simulink model "offboard_SSC_simscape"  (R2025b)
settings: Solver=ode23t  StartTime=0.0  StopTime=0.5  RelTol=1e-3
undefined symbols (not defined in the file): PLL_3ph__class, V_ref
libraries: fl_lib x43, nesl_utility x23, ee_lib x9, simulink x6, eeTransforms x2, batteryecm_lib x1, eeSinusoidalMeasurement x1
(part 2 of 2)

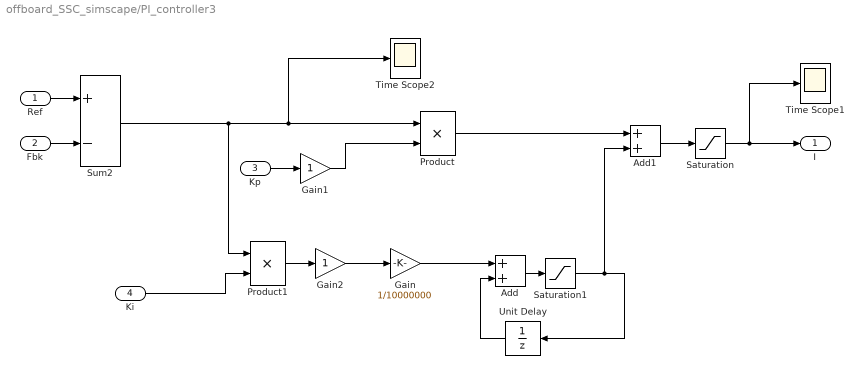
== system offboard_SSC_simscape/PI_controller3 ==
  Ref : Inport
  Fbk : Inport  Port=2
  Kp : Inport  Port=3
  Ki : Inport  Port=4
  Add : Sum
  Add1 : Sum
  Gain : Gain  Gain=1/10000000
  Gain1 : Gain
  Gain2 : Gain
  Product : Product  OutDataTypeStr=Inherit: Same as first input
  Product1 : Product  OutDataTypeStr=Inherit: Same as first input
  Saturation : Saturate  UpperLimit=50  LowerLimit=-50  LinearizeAsGain=off  ZeroCross=off
  Saturation1 : Saturate  UpperLimit=50  LowerLimit=-50  LinearizeAsGain=off  ZeroCross=off
  Sum2 : Sum  Inputs=+-
  Time Scope1 : Scope
      settings: TimeUnits=Metric (based on Time Span)  ActiveDisplayYMinimum=10.50458  ActiveDisplayYMaximum=21.05505  YLabel=Amplitude  DataLoggingVariableName=ScopeData5
  Time Scope2 : Scope
      settings: TimeUnits=Metric (based on Time Span)  ActiveDisplayYMinimum=-48.22028  ActiveDisplayYMaximum=227.58003  YLabel=Amplitude  DataLoggingVariableName=ScopeData6
  Unit Delay : UnitDelay  InitialCondition=0.9  SampleTime=-1  HasFrameUpgradeWarning=on
  I : Outport
  wires:
  Fbk/1 -> Sum2/2
  Ref/1 -> Sum2/1
  Product1/1 -> Gain2/1
  Product/1 -> Add1/1
  Gain/1 -> Add/1
  Unit Delay/1 -> Add/2
  Ki/1 -> Product1/2
  Gain2/1 -> Gain/1
  Add1/1 -> Saturation/1
  Saturation/1 -> Time Scope1/1, I/1
  Kp/1 -> Gain1/1
  Gain1/1 -> Product/2
  Sum2/1 -> Product1/1, Time Scope2/1, Product/1
  Add/1 -> Saturation1/1
  Saturation1/1 -> Add1/2, Unit Delay/1

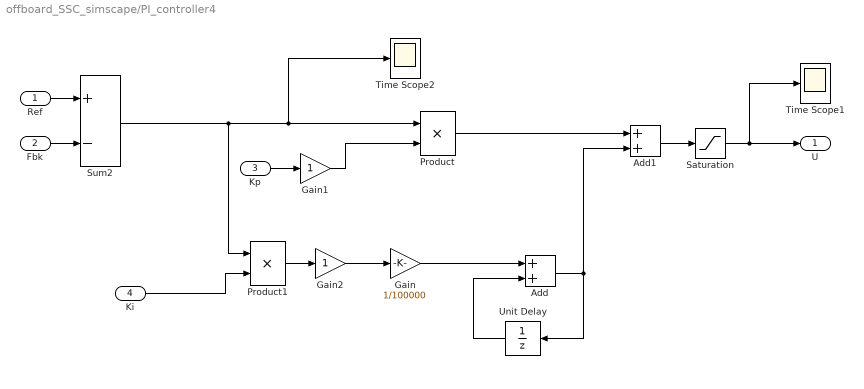
== system offboard_SSC_simscape/PI_controller4 ==
  Ref : Inport
  Fbk : Inport  Port=2
  Kp : Inport  Port=3
  Ki : Inport  Port=4
  Add : Sum
  Add1 : Sum
  Gain : Gain  Gain=1/100000
  Gain1 : Gain
  Gain2 : Gain
  Product : Product  OutDataTypeStr=Inherit: Same as first input
  Product1 : Product  OutDataTypeStr=Inherit: Same as first input
  Saturation : Saturate  UpperLimit=400  LowerLimit=-400  LinearizeAsGain=off  ZeroCross=off
  Sum2 : Sum  Inputs=+-
  Time Scope1 : Scope
      settings: TimeUnits=Metric (based on Time Span)  ActiveDisplayYMinimum=-500  ActiveDisplayYMaximum=500  YLabel=Amplitude  DataLoggingVariableName=ScopeData5
  Time Scope2 : Scope
      settings: TimeUnits=Metric (based on Time Span)  ActiveDisplayYMinimum=-48.22028  ActiveDisplayYMaximum=227.58003  YLabel=Amplitude  DataLoggingVariableName=ScopeData6
  Unit Delay : UnitDelay  SampleTime=-1  HasFrameUpgradeWarning=on
  U : Outport
  wires:
  Fbk/1 -> Sum2/2
  Ref/1 -> Sum2/1
  Product1/1 -> Gain2/1
  Add/1 -> Unit Delay/1, Add1/2
  Product/1 -> Add1/1
  Gain/1 -> Add/1
  Unit Delay/1 -> Add/2
  Ki/1 -> Product1/2
  Gain2/1 -> Gain/1
  Add1/1 -> Saturation/1
  Saturation/1 -> Time Scope1/1, U/1
  Kp/1 -> Gain1/1
  Gain1/1 -> Product/2
  Sum2/1 -> Product1/1, Time Scope2/1, Product/1

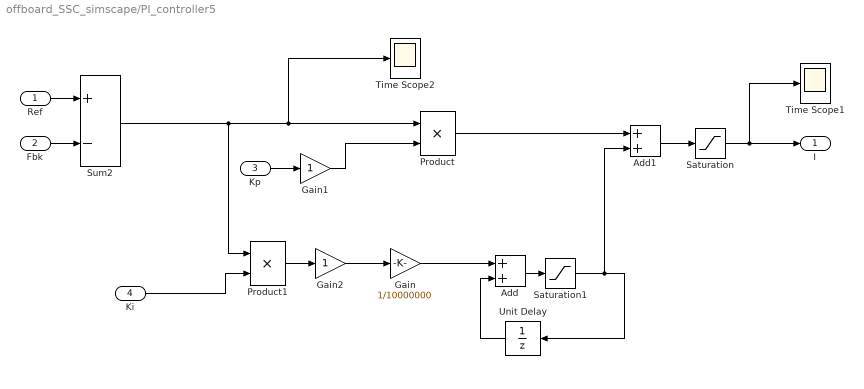
== system offboard_SSC_simscape/PI_controller5 ==
  Ref : Inport
  Fbk : Inport  Port=2
  Kp : Inport  Port=3
  Ki : Inport  Port=4
  Add : Sum
  Add1 : Sum
  Gain : Gain  Gain=1/10000000
  Gain1 : Gain
  Gain2 : Gain
  Product : Product  OutDataTypeStr=Inherit: Same as first input
  Product1 : Product  OutDataTypeStr=Inherit: Same as first input
  Saturation : Saturate  UpperLimit=50  LowerLimit=0  LinearizeAsGain=off  ZeroCross=off
  Saturation1 : Saturate  UpperLimit=50  LowerLimit=-50  LinearizeAsGain=off  ZeroCross=off
  Sum2 : Sum  Inputs=+-
  Time Scope1 : Scope
      settings: TimeUnits=Metric (based on Time Span)  ActiveDisplayYMinimum=10.50458  ActiveDisplayYMaximum=21.05505  YLabel=Amplitude  DataLoggingVariableName=ScopeData5
  Time Scope2 : Scope
      settings: TimeUnits=Metric (based on Time Span)  ActiveDisplayYMinimum=-48.22028  ActiveDisplayYMaximum=227.58003  YLabel=Amplitude  DataLoggingVariableName=ScopeData6
  Unit Delay : UnitDelay  InitialCondition=0.9  SampleTime=-1  HasFrameUpgradeWarning=on
  I : Outport
  wires:
  Fbk/1 -> Sum2/2
  Ref/1 -> Sum2/1
  Product1/1 -> Gain2/1
  Product/1 -> Add1/1
  Gain/1 -> Add/1
  Unit Delay/1 -> Add/2
  Ki/1 -> Product1/2
  Gain2/1 -> Gain/1
  Add1/1 -> Saturation/1
  Saturation/1 -> Time Scope1/1, I/1
  Kp/1 -> Gain1/1
  Gain1/1 -> Product/2
  Sum2/1 -> Product1/1, Time Scope2/1, Product/1
  Add/1 -> Saturation1/1
  Saturation1/1 -> Add1/2, Unit Delay/1

== system offboard_SSC_simscape/PLL (3ph) ==
  abc : Inport
  "Sinusoidal Measurement (PLL, Three-Phase)" : eeSinusoidalMeasurement/Sinusoidal Measurement (PLL, Three-Phase)  Kp_LF=180  Ki_LF=3200  F0=60  Theta0=PLL_3ph__class([0 60]).objParamMappingDerived.NewDerivedParam.Theta0  Ts=0.0001
  Terminator : Terminator
  Freq : Outport  VectorParamsAs1DForOutWhenUnconnected=off
  wt : Outport  Port=2  VectorParamsAs1DForOutWhenUnconnected=off
  wires:
  "Sinusoidal Measurement (PLL, Three-Phase)"/3 -> Terminator/1
  "Sinusoidal Measurement (PLL, Three-Phase)"/2 -> wt/1
  "Sinusoidal Measurement (PLL, Three-Phase)"/1 -> Freq/1
  abc/1 -> "Sinusoidal Measurement (PLL, Three-Phase)"/1

== system offboard_SSC_simscape/Subsystem ==
  PS-Simulink Converter2 : nesl_utility/PS-Simulink Converter  PhysicalDomain=network_engine_domain  SubClassName=ps_output  LeftPortType=input  RightPortType=output  PseudoPeriodic=off  Frequencies=[]  VectorFormat=inherit  Unit=inherit  AffineConversion=off
  Unit Delay1 : UnitDelay  SampleTime=-1  HasFrameUpgradeWarning=on
  Voltage Sensor : fl_lib/Electrical/Electrical Sensors/Voltage Sensor
  + : PMIOPort  Side=Left
  - : PMIOPort  Port=2  Side=Right
  V : Outport
  wires:
  PS-Simulink Converter2/1 -> Unit Delay1/1
  Unit Delay1/1 -> V/1
  connections:
  Voltage Sensor/LConn1 -- +/RConn1
  PS-Simulink Converter2/LConn1 -- Voltage Sensor/RConn1
  Voltage Sensor/RConn2 -- -/RConn1

== system offboard_SSC_simscape/Subsystem1 ==
  Va : Inport
  Va1 : Inport  Port=2
  Add1 : Sum
  Constant8 : Constant  Value=0.5
  Divide : Product  Inputs=*/
  Logical Operator1 : Logic  Operator=NOT  AllPortsSameDT=off  OutDataTypeStr=boolean
  Relational Operator : RelationalOperator  OutDataTypeStr=boolean  ZeroCross=off  InputSameDT=off
  Repeating Sequence : simulink/Sources/Repeating Sequence  rep_seq_t=[0 1/30000/2 1/30000]  rep_seq_y=[0 1 0]
  Scope1 : Scope  NumInputPorts=2
      settings: ActiveDisplayYMinimum=-0.12496  ActiveDisplayYMaximum=1.12466  DataLoggingVariableName=ScopeData3
  Scope2 : Scope  NumInputPorts=2
      settings: ActiveDisplayYMinimum=-0.59999  ActiveDisplayYMaximum=3.15933
  Scope3 : Scope  NumInputPorts=2
      settings: ActiveDisplayYMinimum=-0.125  ActiveDisplayYMaximum=1.125  DataLoggingVariableName=ScopeData2
  Vcomp*2 : Constant  Value=1200
  A : Outport
  A' : Outport  Port=2
  wires:
  Va/1 -> Divide/1
  Divide/1 -> Add1/1
  Add1/1 -> Scope2/1, Relational Operator/2
  Constant8/1 -> Add1/2
  Repeating Sequence/1 -> Scope1/1, Relational Operator/1
  Logical Operator1/1 -> Scope3/1, A/1
  Relational Operator/1 -> Scope3/2, A'/1, Logical Operator1/1
  Va1/1 -> Divide/2

== system offboard_SSC_simscape/Subsystem2 ==
  Vb : Inport
  Va : Inport  Port=2
  Add1 : Sum
  Constant8 : Constant  Value=0.5
  Divide : Product  Inputs=*/
  Logical Operator1 : Logic  Operator=NOT  AllPortsSameDT=off  OutDataTypeStr=boolean
  Relational Operator : RelationalOperator  OutDataTypeStr=boolean  ZeroCross=off  InputSameDT=off
  Repeating Sequence : simulink/Sources/Repeating Sequence  rep_seq_t=[0 1/30000/2 1/30000]  rep_seq_y=[0 1 0]
  Scope1 : Scope  NumInputPorts=2
      settings: ActiveDisplayYMinimum=-0.125  ActiveDisplayYMaximum=1.125  DataLoggingVariableName=ScopeData3
  Scope4 : Scope  NumInputPorts=2
      settings: ActiveDisplayYMinimum=-500  ActiveDisplayYMaximum=500  DataLoggingVariableName=ScopeData3
  Vcomp*2 : Constant  Value=1200
  B : Outport
  B' : Outport  Port=2
  wires:
  Vb/1 -> Divide/1
  Divide/1 -> Add1/1
  Add1/1 -> Relational Operator/2, Scope4/2
  Constant8/1 -> Add1/2
  Repeating Sequence/1 -> Scope1/1, Relational Operator/1
  Logical Operator1/1 -> B/1
  Relational Operator/1 -> B'/1, Logical Operator1/1
  Va/1 -> Divide/2

== system offboard_SSC_simscape/Subsystem3 ==
  Va : Inport
  Add1 : Sum
  Constant8 : Constant  Value=0.5
  Divide : Product  Inputs=*/
  Logical Operator1 : Logic  Operator=NOT  AllPortsSameDT=off  OutDataTypeStr=boolean
  Relational Operator : RelationalOperator  OutDataTypeStr=boolean  ZeroCross=off  InputSameDT=off
  Repeating Sequence : simulink/Sources/Repeating Sequence  rep_seq_t=[0 1/100000/2 1/100000]  rep_seq_y=[0 1 0]
  Scope1 : Scope  NumInputPorts=2
      settings: ActiveDisplayYMinimum=-0.12496  ActiveDisplayYMaximum=1.12466  DataLoggingVariableName=ScopeData3
  Scope2 : Scope  NumInputPorts=2
      settings: ActiveDisplayYMinimum=-0.59999  ActiveDisplayYMaximum=3.15933
  Scope3 : Scope  NumInputPorts=2
      settings: ActiveDisplayYMinimum=-0.125  ActiveDisplayYMaximum=1.125  DataLoggingVariableName=ScopeData2
  Vcomp*2 : Constant  Value=800
  A : Outport
  A' : Outport  Port=2
  wires:
  Va/1 -> Divide/1
  Divide/1 -> Add1/1
  Add1/1 -> Scope2/1, Relational Operator/2
  Constant8/1 -> Add1/2
  Repeating Sequence/1 -> Scope1/1, Relational Operator/1
  Logical Operator1/1 -> Scope3/1, A/1
  Relational Operator/1 -> Scope3/2, A'/1, Logical Operator1/1
  Vcomp*2/1 -> Divide/2

== system offboard_SSC_simscape/Subsystem4 ==
  Vc : Inport
  Va : Inport  Port=2
  Add1 : Sum
  Constant8 : Constant  Value=0.5
  Divide : Product  Inputs=*/
  Logical Operator1 : Logic  Operator=NOT  AllPortsSameDT=off  OutDataTypeStr=boolean
  Relational Operator : RelationalOperator  OutDataTypeStr=boolean  ZeroCross=off  InputSameDT=off
  Repeating Sequence : simulink/Sources/Repeating Sequence  rep_seq_t=[0 1/30000/2 1/30000]  rep_seq_y=[0 1 0]
  Scope1 : Scope  NumInputPorts=2
      settings: ActiveDisplayYMinimum=-0.125  ActiveDisplayYMaximum=1.125  DataLoggingVariableName=ScopeData3
  Scope4 : Scope  NumInputPorts=2
      settings: ActiveDisplayYMinimum=-500  ActiveDisplayYMaximum=500  DataLoggingVariableName=ScopeData3
  Vcomp*2 : Constant  Value=1200
  C : Outport
  C' : Outport  Port=2
  wires:
  Vc/1 -> Divide/1
  Divide/1 -> Add1/1
  Add1/1 -> Relational Operator/2, Scope4/2
  Constant8/1 -> Add1/2
  Repeating Sequence/1 -> Scope1/1, Relational Operator/1
  Logical Operator1/1 -> C/1
  Relational Operator/1 -> C'/1, Logical Operator1/1
  Va/1 -> Divide/2

== system offboard_SSC_simscape/Subsystem5 ==
  Va : Inport
  Add1 : Sum
  Constant8 : Constant  Value=0.5
  Divide : Product  Inputs=*/
  Logical Operator1 : Logic  Operator=NOT  AllPortsSameDT=off  OutDataTypeStr=boolean
  Relational Operator : RelationalOperator  OutDataTypeStr=boolean  ZeroCross=off  InputSameDT=off
  Repeating Sequence : simulink/Sources/Repeating Sequence  rep_seq_t=[0 1/100000/2 1/100000]  rep_seq_y=[0 1 0]
  Scope1 : Scope  NumInputPorts=2
      settings: ActiveDisplayYMinimum=-0.12496  ActiveDisplayYMaximum=1.12466  DataLoggingVariableName=ScopeData3
  Scope2 : Scope  NumInputPorts=2
      settings: ActiveDisplayYMinimum=-0.59999  ActiveDisplayYMaximum=3.15933
  Scope3 : Scope  NumInputPorts=2
      settings: ActiveDisplayYMinimum=-0.125  ActiveDisplayYMaximum=1.125  DataLoggingVariableName=ScopeData2
  Vcomp*2 : Constant  Value=800
  A : Outport
  A' : Outport  Port=2
  wires:
  Va/1 -> Divide/1
  Divide/1 -> Add1/1
  Add1/1 -> Scope2/1, Relational Operator/2
  Constant8/1 -> Add1/2
  Repeating Sequence/1 -> Scope1/1, Relational Operator/1
  Logical Operator1/1 -> Scope3/1, A/1
  Relational Operator/1 -> Scope3/2, A'/1, Logical Operator1/1
  Vcomp*2/1 -> Divide/2

== system offboard_SSC_simscape/Subsystem6 ==
  Va : Inport
  Add1 : Sum
  Constant8 : Constant  Value=0.5
  Divide : Product  Inputs=*/
  Logical Operator1 : Logic  Operator=NOT  AllPortsSameDT=off  OutDataTypeStr=boolean
  Relational Operator : RelationalOperator  OutDataTypeStr=boolean  ZeroCross=off  InputSameDT=off
  Repeating Sequence : simulink/Sources/Repeating Sequence  rep_seq_t=[0 1/100000/2 1/100000]  rep_seq_y=[0 1 0]
  Scope1 : Scope  NumInputPorts=2
      settings: ActiveDisplayYMinimum=-0.12496  ActiveDisplayYMaximum=1.12466  DataLoggingVariableName=ScopeData3
  Scope2 : Scope  NumInputPorts=2
      settings: ActiveDisplayYMinimum=-0.59999  ActiveDisplayYMaximum=3.15933
  Scope3 : Scope  NumInputPorts=2
      settings: ActiveDisplayYMinimum=-0.125  ActiveDisplayYMaximum=1.125  DataLoggingVariableName=ScopeData2
  Vcomp*2 : Constant  Value=800
  A : Outport
  A' : Outport  Port=2
  wires:
  Va/1 -> Divide/1
  Divide/1 -> Add1/1
  Add1/1 -> Scope2/1, Relational Operator/2
  Constant8/1 -> Add1/2
  Repeating Sequence/1 -> Scope1/1, Relational Operator/1
  Logical Operator1/1 -> Scope3/1, A/1
  Relational Operator/1 -> Scope3/2, A'/1, Logical Operator1/1
  Vcomp*2/1 -> Divide/2

== system offboard_SSC_simscape/Subsystem8 ==
  PS-Simulink Converter2 : nesl_utility/PS-Simulink Converter  PhysicalDomain=network_engine_domain  SubClassName=ps_output  LeftPortType=input  RightPortType=output  PseudoPeriodic=off  Frequencies=[]  VectorFormat=inherit  Unit=inherit  AffineConversion=off
  Unit Delay1 : UnitDelay  SampleTime=-1  HasFrameUpgradeWarning=on
  Voltage Sensor : fl_lib/Electrical/Electrical Sensors/Voltage Sensor
  + : PMIOPort  Side=Left
  - : PMIOPort  Port=2  Side=Right
  V : Outport
  wires:
  Unit Delay1/1 -> V/1
  PS-Simulink Converter2/1 -> Unit Delay1/1
  connections:
  Voltage Sensor/RConn2 -- -/RConn1
  PS-Simulink Converter2/LConn1 -- Voltage Sensor/RConn1
  Voltage Sensor/LConn1 -- +/RConn1

== system offboard_SSC_simscape/DC//DC1/S1 ==
  g : Inport
  Diode : fl_lib/Electrical/Electrical Elements/Diode  Vf=1e-3 V  Ron=1e-2 Ohm  Goff=1e-5 1/Ohm  i_specify=off  i_priority=None  i=0 A  i_nominal_specify=off  i_nominal_value=1  i_nominal_unit=A  v_specify=off  v_priority=None  v=0 V  v_nominal_specify=off  v_nominal_value=1  v_nominal_unit=V
  S1 : fl_lib/Electrical/Electrical Elements/Switch  R_closed=0.1 Ohm  G_open=1e-5 1/Ohm  Threshold=0.5  i_specify=off  i_priority=None  i=0 A  i_nominal_specify=off  i_nominal_value=1  i_nominal_unit=A  v_specify=off  v_priority=None  v=0 V  v_nominal_specify=off  v_nominal_value=1  v_nominal_unit=V
  Simulink-PS Converter : nesl_utility/Simulink-PS Converter  PhysicalDomain=network_engine_domain  SubClassName=ps_input  LeftPortType=input  RightPortType=output  PseudoPeriodic=off  Frequencies=[]  NoiseDistribution=none  NoiseParameters=[]  Unit=1  AffineConversion=off  FilteringAndDerivatives=zero  SimscapeFilterOrder=1  InputFilterTimeConstant=0.001  UdotUserProvided=0
  + : PMIOPort  Side=Left
  - : PMIOPort  Port=2  Side=Right
  wires:
  g/1 -> Simulink-PS Converter/1
  connections:
  S1/RConn2 -- -/RConn1 -- Diode/LConn1
  Diode/RConn1 -- +/RConn1 -- S1/LConn1
  Simulink-PS Converter/RConn1 -- S1/RConn1

== system offboard_SSC_simscape/DC//DC1/S2 ==
  g : Inport
  Diode : fl_lib/Electrical/Electrical Elements/Diode  Vf=1e-3 V  Ron=1e-2 Ohm  Goff=1e-5 1/Ohm  i_specify=off  i_priority=None  i=0 A  i_nominal_specify=off  i_nominal_value=1  i_nominal_unit=A  v_specify=off  v_priority=None  v=0 V  v_nominal_specify=off  v_nominal_value=1  v_nominal_unit=V
  S1 : fl_lib/Electrical/Electrical Elements/Switch  R_closed=0.1 Ohm  G_open=1e-5 1/Ohm  Threshold=0.5  i_specify=off  i_priority=None  i=0 A  i_nominal_specify=off  i_nominal_value=1  i_nominal_unit=A  v_specify=off  v_priority=None  v=0 V  v_nominal_specify=off  v_nominal_value=1  v_nominal_unit=V
  Simulink-PS Converter : nesl_utility/Simulink-PS Converter  PhysicalDomain=network_engine_domain  SubClassName=ps_input  LeftPortType=input  RightPortType=output  PseudoPeriodic=off  Frequencies=[]  NoiseDistribution=none  NoiseParameters=[]  Unit=1  AffineConversion=off  FilteringAndDerivatives=zero  SimscapeFilterOrder=1  InputFilterTimeConstant=0.001  UdotUserProvided=0
  + : PMIOPort  Side=Left
  - : PMIOPort  Port=2  Side=Right
  wires:
  g/1 -> Simulink-PS Converter/1
  connections:
  Simulink-PS Converter/RConn1 -- S1/RConn1
  S1/LConn1 -- +/RConn1 -- Diode/RConn1
  Diode/LConn1 -- -/RConn1 -- S1/RConn2

== system offboard_SSC_simscape/DC//DC2/S1 ==
  g : Inport
  Diode : fl_lib/Electrical/Electrical Elements/Diode  Vf=1e-3 V  Ron=1e-2 Ohm  Goff=1e-5 1/Ohm  i_specify=off  i_priority=None  i=0 A  i_nominal_specify=off  i_nominal_value=1  i_nominal_unit=A  v_specify=off  v_priority=None  v=0 V  v_nominal_specify=off  v_nominal_value=1  v_nominal_unit=V
  S1 : fl_lib/Electrical/Electrical Elements/Switch  R_closed=0.1 Ohm  G_open=1e-5 1/Ohm  Threshold=0.5  i_specify=off  i_priority=None  i=0 A  i_nominal_specify=off  i_nominal_value=1  i_nominal_unit=A  v_specify=off  v_priority=None  v=0 V  v_nominal_specify=off  v_nominal_value=1  v_nominal_unit=V
  Simulink-PS Converter : nesl_utility/Simulink-PS Converter  PhysicalDomain=network_engine_domain  SubClassName=ps_input  LeftPortType=input  RightPortType=output  PseudoPeriodic=off  Frequencies=[]  NoiseDistribution=none  NoiseParameters=[]  Unit=1  AffineConversion=off  FilteringAndDerivatives=zero  SimscapeFilterOrder=1  InputFilterTimeConstant=0.001  UdotUserProvided=0
  + : PMIOPort  Side=Left
  - : PMIOPort  Port=2  Side=Right
  wires:
  g/1 -> Simulink-PS Converter/1
  connections:
  S1/RConn2 -- -/RConn1 -- Diode/LConn1
  Diode/RConn1 -- +/RConn1 -- S1/LConn1
  Simulink-PS Converter/RConn1 -- S1/RConn1

== system offboard_SSC_simscape/DC//DC2/S2 ==
  g : Inport
  Diode : fl_lib/Electrical/Electrical Elements/Diode  Vf=1e-3 V  Ron=1e-2 Ohm  Goff=1e-5 1/Ohm  i_specify=off  i_priority=None  i=0 A  i_nominal_specify=off  i_nominal_value=1  i_nominal_unit=A  v_specify=off  v_priority=None  v=0 V  v_nominal_specify=off  v_nominal_value=1  v_nominal_unit=V
  S1 : fl_lib/Electrical/Electrical Elements/Switch  R_closed=0.1 Ohm  G_open=1e-5 1/Ohm  Threshold=0.5  i_specify=off  i_priority=None  i=0 A  i_nominal_specify=off  i_nominal_value=1  i_nominal_unit=A  v_specify=off  v_priority=None  v=0 V  v_nominal_specify=off  v_nominal_value=1  v_nominal_unit=V
  Simulink-PS Converter : nesl_utility/Simulink-PS Converter  PhysicalDomain=network_engine_domain  SubClassName=ps_input  LeftPortType=input  RightPortType=output  PseudoPeriodic=off  Frequencies=[]  NoiseDistribution=none  NoiseParameters=[]  Unit=1  AffineConversion=off  FilteringAndDerivatives=zero  SimscapeFilterOrder=1  InputFilterTimeConstant=0.001  UdotUserProvided=0
  + : PMIOPort  Side=Left
  - : PMIOPort  Port=2  Side=Right
  wires:
  g/1 -> Simulink-PS Converter/1
  connections:
  Simulink-PS Converter/RConn1 -- S1/RConn1
  S1/LConn1 -- +/RConn1 -- Diode/RConn1
  Diode/LConn1 -- -/RConn1 -- S1/RConn2

== system offboard_SSC_simscape/DC//DC3/S1 ==
  g : Inport
  Diode : fl_lib/Electrical/Electrical Elements/Diode  Vf=1e-3 V  Ron=1e-2 Ohm  Goff=1e-5 1/Ohm  i_specify=off  i_priority=None  i=0 A  i_nominal_specify=off  i_nominal_value=1  i_nominal_unit=A  v_specify=off  v_priority=None  v=0 V  v_nominal_specify=off  v_nominal_value=1  v_nominal_unit=V
  S1 : fl_lib/Electrical/Electrical Elements/Switch  R_closed=0.1 Ohm  G_open=1e-5 1/Ohm  Threshold=0.5  i_specify=off  i_priority=None  i=0 A  i_nominal_specify=off  i_nominal_value=1  i_nominal_unit=A  v_specify=off  v_priority=None  v=0 V  v_nominal_specify=off  v_nominal_value=1  v_nominal_unit=V
  Simulink-PS Converter : nesl_utility/Simulink-PS Converter  PhysicalDomain=network_engine_domain  SubClassName=ps_input  LeftPortType=input  RightPortType=output  PseudoPeriodic=off  Frequencies=[]  NoiseDistribution=none  NoiseParameters=[]  Unit=1  AffineConversion=off  FilteringAndDerivatives=zero  SimscapeFilterOrder=1  InputFilterTimeConstant=0.001  UdotUserProvided=0
  + : PMIOPort  Side=Left
  - : PMIOPort  Port=2  Side=Right
  wires:
  g/1 -> Simulink-PS Converter/1
  connections:
  S1/RConn2 -- -/RConn1 -- Diode/LConn1
  Diode/RConn1 -- +/RConn1 -- S1/LConn1
  Simulink-PS Converter/RConn1 -- S1/RConn1

== system offboard_SSC_simscape/DC//DC3/S2 ==
  g : Inport
  Diode : fl_lib/Electrical/Electrical Elements/Diode  Vf=1e-3 V  Ron=1e-2 Ohm  Goff=1e-5 1/Ohm  i_specify=off  i_priority=None  i=0 A  i_nominal_specify=off  i_nominal_value=1  i_nominal_unit=A  v_specify=off  v_priority=None  v=0 V  v_nominal_specify=off  v_nominal_value=1  v_nominal_unit=V
  S1 : fl_lib/Electrical/Electrical Elements/Switch  R_closed=0.1 Ohm  G_open=1e-5 1/Ohm  Threshold=0.5  i_specify=off  i_priority=None  i=0 A  i_nominal_specify=off  i_nominal_value=1  i_nominal_unit=A  v_specify=off  v_priority=None  v=0 V  v_nominal_specify=off  v_nominal_value=1  v_nominal_unit=V
  Simulink-PS Converter : nesl_utility/Simulink-PS Converter  PhysicalDomain=network_engine_domain  SubClassName=ps_input  LeftPortType=input  RightPortType=output  PseudoPeriodic=off  Frequencies=[]  NoiseDistribution=none  NoiseParameters=[]  Unit=1  AffineConversion=off  FilteringAndDerivatives=zero  SimscapeFilterOrder=1  InputFilterTimeConstant=0.001  UdotUserProvided=0
  + : PMIOPort  Side=Left
  - : PMIOPort  Port=2  Side=Right
  wires:
  g/1 -> Simulink-PS Converter/1
  connections:
  Simulink-PS Converter/RConn1 -- S1/RConn1
  S1/LConn1 -- +/RConn1 -- Diode/RConn1
  Diode/LConn1 -- -/RConn1 -- S1/RConn2

== system offboard_SSC_simscape/Front End/S1 ==
  g : Inport
  Diode : fl_lib/Electrical/Electrical Elements/Diode  Vf=1e-3 V  Ron=1e-2 Ohm  Goff=1e-5 1/Ohm  i_specify=off  i_priority=None  i=0 A  i_nominal_specify=off  i_nominal_value=1  i_nominal_unit=A  v_specify=off  v_priority=None  v=0 V  v_nominal_specify=off  v_nominal_value=1  v_nominal_unit=V
  S1 : fl_lib/Electrical/Electrical Elements/Switch  R_closed=0.1 Ohm  G_open=1e-5 1/Ohm  Threshold=0.5  i_specify=off  i_priority=None  i=0 A  i_nominal_specify=off  i_nominal_value=1  i_nominal_unit=A  v_specify=off  v_priority=None  v=0 V  v_nominal_specify=off  v_nominal_value=1  v_nominal_unit=V
  Simulink-PS Converter : nesl_utility/Simulink-PS Converter  PhysicalDomain=network_engine_domain  SubClassName=ps_input  LeftPortType=input  RightPortType=output  PseudoPeriodic=off  Frequencies=[]  NoiseDistribution=none  NoiseParameters=[]  Unit=1  AffineConversion=off  FilteringAndDerivatives=zero  SimscapeFilterOrder=1  InputFilterTimeConstant=0.001  UdotUserProvided=0
  + : PMIOPort  Side=Left
  - : PMIOPort  Port=2  Side=Right
  wires:
  g/1 -> Simulink-PS Converter/1
  connections:
  S1/RConn2 -- -/RConn1 -- Diode/LConn1
  Diode/RConn1 -- S1/LConn1 -- +/RConn1
  Simulink-PS Converter/RConn1 -- S1/RConn1

== system offboard_SSC_simscape/Front End/S2 ==
  g : Inport
  Diode : fl_lib/Electrical/Electrical Elements/Diode  Vf=1e-3 V  Ron=1e-2 Ohm  Goff=1e-5 1/Ohm  i_specify=off  i_priority=None  i=0 A  i_nominal_specify=off  i_nominal_value=1  i_nominal_unit=A  v_specify=off  v_priority=None  v=0 V  v_nominal_specify=off  v_nominal_value=1  v_nominal_unit=V
  S1 : fl_lib/Electrical/Electrical Elements/Switch  R_closed=0.1 Ohm  G_open=1e-5 1/Ohm  Threshold=0.5  i_specify=off  i_priority=None  i=0 A  i_nominal_specify=off  i_nominal_value=1  i_nominal_unit=A  v_specify=off  v_priority=None  v=0 V  v_nominal_specify=off  v_nominal_value=1  v_nominal_unit=V
  Simulink-PS Converter : nesl_utility/Simulink-PS Converter  PhysicalDomain=network_engine_domain  SubClassName=ps_input  LeftPortType=input  RightPortType=output  PseudoPeriodic=off  Frequencies=[]  NoiseDistribution=none  NoiseParameters=[]  Unit=1  AffineConversion=off  FilteringAndDerivatives=zero  SimscapeFilterOrder=1  InputFilterTimeConstant=0.001  UdotUserProvided=0
  + : PMIOPort  Side=Left
  - : PMIOPort  Port=2  Side=Right
  wires:
  g/1 -> Simulink-PS Converter/1
  connections:
  Simulink-PS Converter/RConn1 -- S1/RConn1
  S1/LConn1 -- +/RConn1 -- Diode/RConn1
  Diode/LConn1 -- S1/RConn2 -- -/RConn1

== system offboard_SSC_simscape/Front End/S3 ==
  g : Inport
  Diode : fl_lib/Electrical/Electrical Elements/Diode  Vf=1e-3 V  Ron=1e-2 Ohm  Goff=1e-5 1/Ohm  i_specify=off  i_priority=None  i=0 A  i_nominal_specify=off  i_nominal_value=1  i_nominal_unit=A  v_specify=off  v_priority=None  v=0 V  v_nominal_specify=off  v_nominal_value=1  v_nominal_unit=V
  S1 : fl_lib/Electrical/Electrical Elements/Switch  R_closed=0.1 Ohm  G_open=1e-5 1/Ohm  Threshold=0.5  i_specify=off  i_priority=None  i=0 A  i_nominal_specify=off  i_nominal_value=1  i_nominal_unit=A  v_specify=off  v_priority=None  v=0 V  v_nominal_specify=off  v_nominal_value=1  v_nominal_unit=V
  Simulink-PS Converter : nesl_utility/Simulink-PS Converter  PhysicalDomain=network_engine_domain  SubClassName=ps_input  LeftPortType=input  RightPortType=output  PseudoPeriodic=off  Frequencies=[]  NoiseDistribution=none  NoiseParameters=[]  Unit=1  AffineConversion=off  FilteringAndDerivatives=zero  SimscapeFilterOrder=1  InputFilterTimeConstant=0.001  UdotUserProvided=0
  + : PMIOPort  Side=Left
  - : PMIOPort  Port=2  Side=Right
  wires:
  g/1 -> Simulink-PS Converter/1
  connections:
  -/RConn1 -- S1/RConn2 -- Diode/LConn1
  Diode/RConn1 -- +/RConn1 -- S1/LConn1
  Simulink-PS Converter/RConn1 -- S1/RConn1

== system offboard_SSC_simscape/Front End/S4 ==
  g : Inport
  Diode : fl_lib/Electrical/Electrical Elements/Diode  Vf=1e-3 V  Ron=1e-2 Ohm  Goff=1e-5 1/Ohm  i_specify=off  i_priority=None  i=0 A  i_nominal_specify=off  i_nominal_value=1  i_nominal_unit=A  v_specify=off  v_priority=None  v=0 V  v_nominal_specify=off  v_nominal_value=1  v_nominal_unit=V
  S1 : fl_lib/Electrical/Electrical Elements/Switch  R_closed=0.1 Ohm  G_open=1e-5 1/Ohm  Threshold=0.5  i_specify=off  i_priority=None  i=0 A  i_nominal_specify=off  i_nominal_value=1  i_nominal_unit=A  v_specify=off  v_priority=None  v=0 V  v_nominal_specify=off  v_nominal_value=1  v_nominal_unit=V
  Simulink-PS Converter : nesl_utility/Simulink-PS Converter  PhysicalDomain=network_engine_domain  SubClassName=ps_input  LeftPortType=input  RightPortType=output  PseudoPeriodic=off  Frequencies=[]  NoiseDistribution=none  NoiseParameters=[]  Unit=1  AffineConversion=off  FilteringAndDerivatives=zero  SimscapeFilterOrder=1  InputFilterTimeConstant=0.001  UdotUserProvided=0
  + : PMIOPort  Side=Left
  - : PMIOPort  Port=2  Side=Right
  wires:
  g/1 -> Simulink-PS Converter/1
  connections:
  Simulink-PS Converter/RConn1 -- S1/RConn1
  S1/LConn1 -- +/RConn1 -- Diode/RConn1
  Diode/LConn1 -- S1/RConn2 -- -/RConn1

== system offboard_SSC_simscape/Front End/S5 ==
  g : Inport
  Diode : fl_lib/Electrical/Electrical Elements/Diode  Vf=1e-3 V  Ron=1e-2 Ohm  Goff=1e-5 1/Ohm  i_specify=off  i_priority=None  i=0 A  i_nominal_specify=off  i_nominal_value=1  i_nominal_unit=A  v_specify=off  v_priority=None  v=0 V  v_nominal_specify=off  v_nominal_value=1  v_nominal_unit=V
  S1 : fl_lib/Electrical/Electrical Elements/Switch  R_closed=0.1 Ohm  G_open=1e-5 1/Ohm  Threshold=0.5  i_specify=off  i_priority=None  i=0 A  i_nominal_specify=off  i_nominal_value=1  i_nominal_unit=A  v_specify=off  v_priority=None  v=0 V  v_nominal_specify=off  v_nominal_value=1  v_nominal_unit=V
  Simulink-PS Converter : nesl_utility/Simulink-PS Converter  PhysicalDomain=network_engine_domain  SubClassName=ps_input  LeftPortType=input  RightPortType=output  PseudoPeriodic=off  Frequencies=[]  NoiseDistribution=none  NoiseParameters=[]  Unit=1  AffineConversion=off  FilteringAndDerivatives=zero  SimscapeFilterOrder=1  InputFilterTimeConstant=0.001  UdotUserProvided=0
  + : PMIOPort  Side=Left
  - : PMIOPort  Port=2  Side=Right
  wires:
  g/1 -> Simulink-PS Converter/1
  connections:
  -/RConn1 -- S1/RConn2 -- Diode/LConn1
  Diode/RConn1 -- +/RConn1 -- S1/LConn1
  Simulink-PS Converter/RConn1 -- S1/RConn1

== system offboard_SSC_simscape/Front End/S6 ==
  g : Inport
  Diode : fl_lib/Electrical/Electrical Elements/Diode  Vf=1e-3 V  Ron=1e-2 Ohm  Goff=1e-5 1/Ohm  i_specify=off  i_priority=None  i=0 A  i_nominal_specify=off  i_nominal_value=1  i_nominal_unit=A  v_specify=off  v_priority=None  v=0 V  v_nominal_specify=off  v_nominal_value=1  v_nominal_unit=V
  S1 : fl_lib/Electrical/Electrical Elements/Switch  R_closed=0.1 Ohm  G_open=1e-5 1/Ohm  Threshold=0.5  i_specify=off  i_priority=None  i=0 A  i_nominal_specify=off  i_nominal_value=1  i_nominal_unit=A  v_specify=off  v_priority=None  v=0 V  v_nominal_specify=off  v_nominal_value=1  v_nominal_unit=V
  Simulink-PS Converter : nesl_utility/Simulink-PS Converter  PhysicalDomain=network_engine_domain  SubClassName=ps_input  LeftPortType=input  RightPortType=output  PseudoPeriodic=off  Frequencies=[]  NoiseDistribution=none  NoiseParameters=[]  Unit=1  AffineConversion=off  FilteringAndDerivatives=zero  SimscapeFilterOrder=1  InputFilterTimeConstant=0.001  UdotUserProvided=0
  + : PMIOPort  Side=Left
  - : PMIOPort  Port=2  Side=Right
  wires:
  g/1 -> Simulink-PS Converter/1
  connections:
  Simulink-PS Converter/RConn1 -- S1/RConn1
  S1/LConn1 -- +/RConn1 -- Diode/RConn1
  Diode/LConn1 -- S1/RConn2 -- -/RConn1
